simulink model "lyap"  (R2016a)
settings: Solver=FixedStepDiscrete  StartTime=0.0  StopTime=10.0  RelTol=1e-3
libraries: rvs x16
settings Model: Creator=Arthur  LastModifiedBy=arthur
settings DataIOCC: LimitDataPoints=on  SaveFormat=Array
settings DebuggingCC: SolverPrmCheckMsg=warning
settings HardwareCC: ProdBitPerPointer=32  ProdLargestAtomicFloat=None  ProdIntDivRoundTo=Undefined  ProdEndianess=Unspecified  ProdWordSize=32  ProdHWDeviceType=32-bit Generic
settings ModelReferenceCC: PropagateSignalLabelsOutOfModel=off
settings ConfigComp: CovModelRefEnable=Off  CovSFcnEnable=off

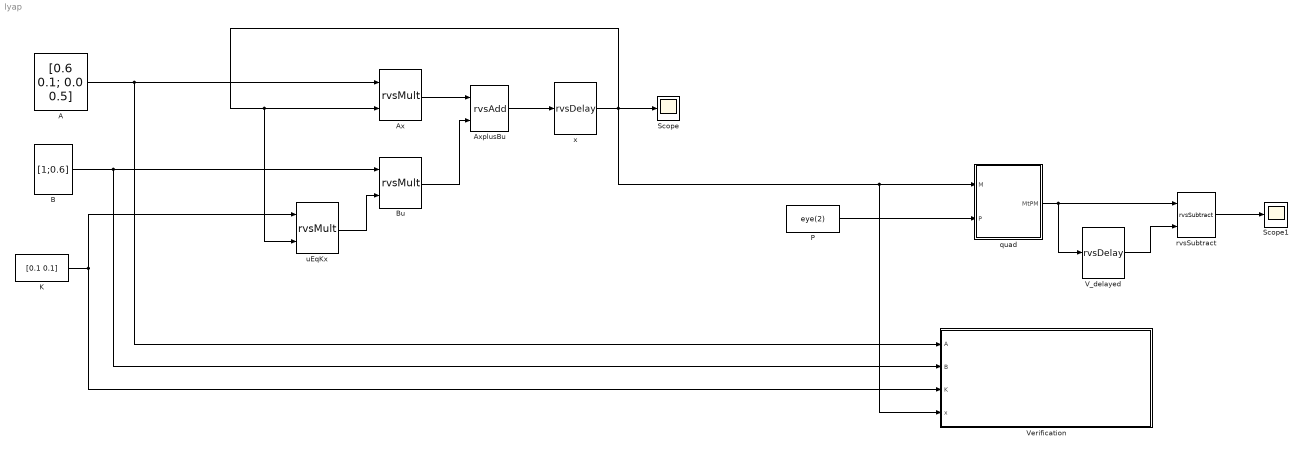
== system lyap ==
  A : Constant  Value=[0.6 0.1; 0.0 0.5]
  Ax : rvs/rvsMult
  AxplusBu : rvs/rvsAdd
  B : Constant  Value=[1;0.6]  VectorParams1D=off
  Bu : rvs/rvsMult
  K : Constant  Value=[0.1 0.1]  VectorParams1D=off
  P : Constant  Value=eye(2)  VectorParams1D=off
  Scope : Scope
  Scope1 : Scope
  V_delayed : rvs/rvsDelay  xInit=0
  Verification : Subsystem
  quad : Subsystem
  rvsSubtract : rvs/rvsSubtract
  uEqKx : rvs/rvsMult
  x : rvs/rvsDelay  xInit=[0.7;-0.5]
  wires:
  Ax/1 -> AxplusBu/1
  Bu/1 -> AxplusBu/2
  uEqKx/1 -> Bu/2
  AxplusBu/1 -> x/1
  A/1 -> Verification/1(A), Ax/1
  B/1 -> Verification/2(B), Bu/1
  x/1 -> Scope/1, quad/1(M), Verification/4(x), uEqKx/2, Ax/2
  K/1 -> Verification/3(K), uEqKx/1
  P/1 -> quad/2(P)
  quad/1(MtPM) -> rvsSubtract/1, V_delayed/1
  V_delayed/1 -> rvsSubtract/2
  rvsSubtract/1 -> Scope1/1

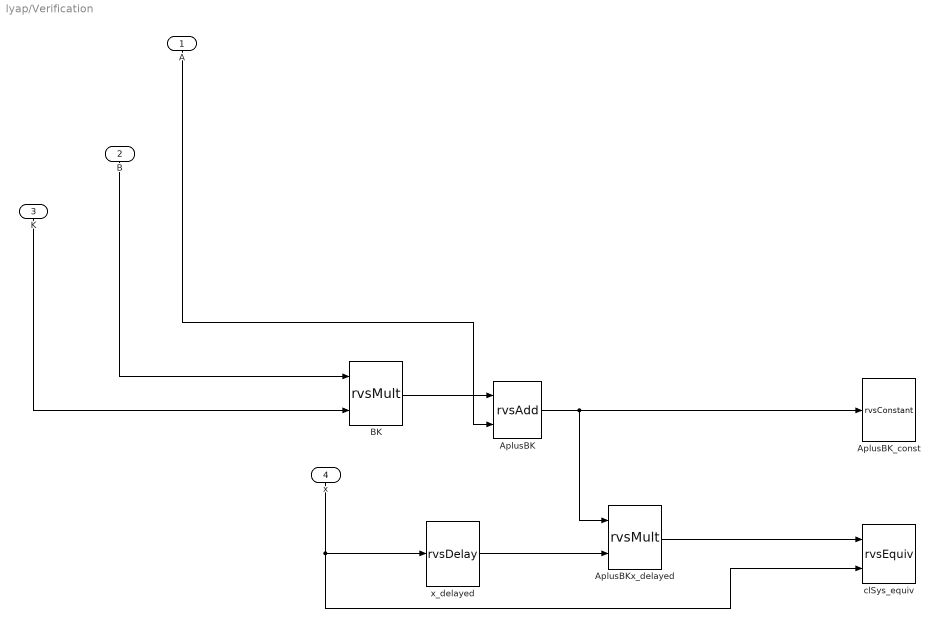
== system lyap/Verification ==
  A : Inport
  B : Inport  Port=2
  K : Inport  Port=3
  x : Inport  Port=4
  AplusBK : rvs/rvsAdd
  AplusBK_const : rvs/rvsConstant
  AplusBKx_delayed : rvs/rvsMult
  BK : rvs/rvsMult
  clSys_equiv : rvs/rvsEquiv  tol=1e-9  nIgnoreSteps=1
  x_delayed : rvs/rvsDelay  xInit=[0]
  wires:
  A/1 -> AplusBK/2
  B/1 -> BK/1
  K/1 -> BK/2
  BK/1 -> AplusBK/1
  AplusBK/1 -> AplusBKx_delayed/1, AplusBK_const/1
  x_delayed/1 -> AplusBKx_delayed/2
  AplusBKx_delayed/1 -> clSys_equiv/1
  x/1 -> clSys_equiv/2, x_delayed/1

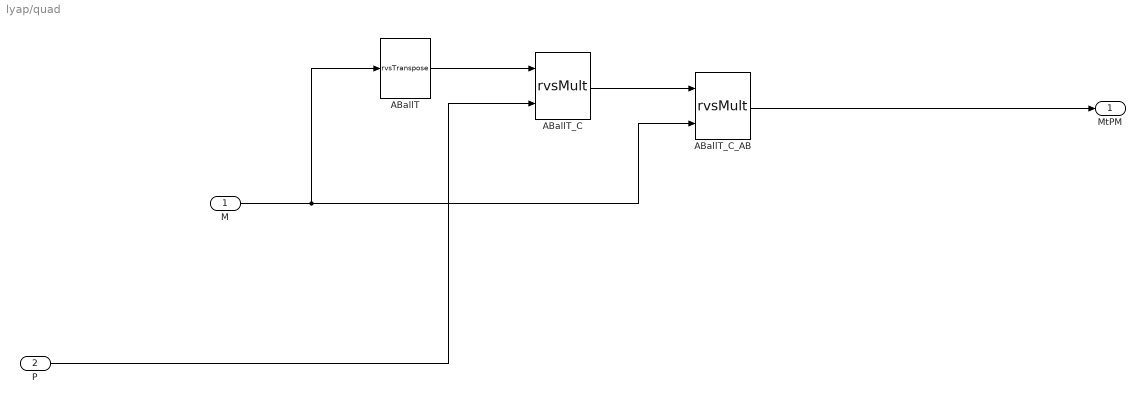
== system lyap/quad ==
  M : Inport
  P : Inport  Port=2
  ABallT : rvs/rvsTranspose
  ABallT_C : rvs/rvsMult
  ABallT_C_AB : rvs/rvsMult
  MtPM : Outport
  wires:
  ABallT_C/1 -> ABallT_C_AB/1
  M/1 -> ABallT/1, ABallT_C_AB/2
  ABallT/1 -> ABallT_C/1
  P/1 -> ABallT_C/2
  ABallT_C_AB/1 -> MtPM/1
